simulink model "nuclearReactor"  (R2014b)
settings: Solver=ode1  StartTime=0.0  StopTime=100  FixedStep=0.0001  MaxStep=0.0001  RelTol=1e-3
(part 4 of 4)

== matlab function nuclearReactor/Controller20/MATLAB Function ==
  data: q input; qNext output; x input; r1 output; r2 output; y1 input; y2 input; control output


function [qNext,r1,r2,control]  = phi(q, x, y1, y2)
%#codegen
% control {-1 undefined, 0 add1, 1 remove1, 2 add2, 3 remove2}

undef =0;
add1 = 1;
remove1 =2;
add2 = 3;
remove2 =4;
c=15;

if q==0 
    %When plant is in T0 ("No Rod")
    if x > 550 && y1 >= c && y2<c
        qNext=1;
        r1=0; r2=0;
        control=add1;
    elseif x>550 && y2>=c
        qNext=2;
        r1=0; r2=0;
        control=add2;
    else
        qNext=0;
        r1=0; r2=0;
        control=undef;
    end;
    
elseif q==1    
    %When plant is in T1 ("Rod One")
    if x <= 510 
        qNext=0;
        r1=1; r2=0;
        control=remove1;
    else
        qNext=1;
        r1=0; r2=0;
        control=undef;
    end;

elseif q==2    
    %When plant is in T2 ("Rod Two")
    if x <= 510 
        qNext=0;
        r1=0; r2=1;
        control=remove2;
    else
        qNext=2;
        r1=0; r2=0;
        control=undef;
    end;
else
    qNext=-1; %this should never execute
    r1=0; r2=0; %this should never execute
    control=-1; %this should never execute
end

== matlab function nuclearReactor/Controller21/MATLAB Function ==
  data: q input; qNext output; x input; r1 output; r2 output; y1 input; y2 input; control output


function [qNext,r1,r2,control]  = phi(q, x, y1, y2)
%#codegen
% control {-1 undefined, 0 add1, 1 remove1, 2 add2, 3 remove2}

undef =0;
add1 = 1;
remove1 =2;
add2 = 3;
remove2 =4;
c=15;

if q==0 
    %When plant is in T0 ("No Rod")
    if x > 550 && y1 >= c && y2<c
        qNext=1;
        r1=0; r2=0;
        control=add1;
    elseif x>550 && y2>=c
        qNext=2;
        r1=0; r2=0;
        control=add2;
    else
        qNext=0;
        r1=0; r2=0;
        control=undef;
    end;
    
elseif q==1    
    %When plant is in T1 ("Rod One")
    if x <= 510 
        qNext=0;
        r1=1; r2=0;
        control=remove1;
    else
        qNext=1;
        r1=0; r2=0;
        control=undef;
    end;

elseif q==2    
    %When plant is in T2 ("Rod Two")
    if x <= 510 
        qNext=0;
        r1=0; r2=1;
        control=remove2;
    else
        qNext=2;
        r1=0; r2=0;
        control=undef;
    end;
else
    qNext=-1; %this should never execute
    r1=0; r2=0; %this should never execute
    control=-1; %this should never execute
end

== matlab function nuclearReactor/Controller22/MATLAB Function ==
  data: q input; qNext output; x input; r1 output; r2 output; y1 input; y2 input; control output


function [qNext,r1,r2,control]  = phi(q, x, y1, y2)
%#codegen
% control {-1 undefined, 0 add1, 1 remove1, 2 add2, 3 remove2}

undef =0;
add1 = 1;
remove1 =2;
add2 = 3;
remove2 =4;
c=15;

if q==0 
    %When plant is in T0 ("No Rod")
    if x > 550 && y1 >= c && y2<c
        qNext=1;
        r1=0; r2=0;
        control=add1;
    elseif x>550 && y2>=c
        qNext=2;
        r1=0; r2=0;
        control=add2;
    else
        qNext=0;
        r1=0; r2=0;
        control=undef;
    end;
    
elseif q==1    
    %When plant is in T1 ("Rod One")
    if x <= 510 
        qNext=0;
        r1=1; r2=0;
        control=remove1;
    else
        qNext=1;
        r1=0; r2=0;
        control=undef;
    end;

elseif q==2    
    %When plant is in T2 ("Rod Two")
    if x <= 510 
        qNext=0;
        r1=0; r2=1;
        control=remove2;
    else
        qNext=2;
        r1=0; r2=0;
        control=undef;
    end;
else
    qNext=-1; %this should never execute
    r1=0; r2=0; %this should never execute
    control=-1; %this should never execute
end

== matlab function nuclearReactor/Controller23/MATLAB Function ==
  data: q input; qNext output; x input; r1 output; r2 output; y1 input; y2 input; control output


function [qNext,r1,r2,control]  = phi(q, x, y1, y2)
%#codegen
% control {-1 undefined, 0 add1, 1 remove1, 2 add2, 3 remove2}

undef =0;
add1 = 1;
remove1 =2;
add2 = 3;
remove2 =4;
c=15;

if q==0 
    %When plant is in T0 ("No Rod")
    if x > 550 && y1 >= c && y2<c
        qNext=1;
        r1=0; r2=0;
        control=add1;
    elseif x>550 && y2>=c
        qNext=2;
        r1=0; r2=0;
        control=add2;
    else
        qNext=0;
        r1=0; r2=0;
        control=undef;
    end;
    
elseif q==1    
    %When plant is in T1 ("Rod One")
    if x <= 510 
        qNext=0;
        r1=1; r2=0;
        control=remove1;
    else
        qNext=1;
        r1=0; r2=0;
        control=undef;
    end;

elseif q==2    
    %When plant is in T2 ("Rod Two")
    if x <= 510 
        qNext=0;
        r1=0; r2=1;
        control=remove2;
    else
        qNext=2;
        r1=0; r2=0;
        control=undef;
    end;
else
    qNext=-1; %this should never execute
    r1=0; r2=0; %this should never execute
    control=-1; %this should never execute
end

== matlab function nuclearReactor/Controller24/MATLAB Function ==
  data: q input; qNext output; x input; r1 output; r2 output; y1 input; y2 input; control output


function [qNext,r1,r2,control]  = phi(q, x, y1, y2)
%#codegen
% control {-1 undefined, 0 add1, 1 remove1, 2 add2, 3 remove2}

undef =0;
add1 = 1;
remove1 =2;
add2 = 3;
remove2 =4;
c=15;

if q==0 
    %When plant is in T0 ("No Rod")
    if x > 550 && y1 >= c && y2<c
        qNext=1;
        r1=0; r2=0;
        control=add1;
    elseif x>550 && y2>=c
        qNext=2;
        r1=0; r2=0;
        control=add2;
    else
        qNext=0;
        r1=0; r2=0;
        control=undef;
    end;
    
elseif q==1    
    %When plant is in T1 ("Rod One")
    if x <= 510 
        qNext=0;
        r1=1; r2=0;
        control=remove1;
    else
        qNext=1;
        r1=0; r2=0;
        control=undef;
    end;

elseif q==2    
    %When plant is in T2 ("Rod Two")
    if x <= 510 
        qNext=0;
        r1=0; r2=1;
        control=remove2;
    else
        qNext=2;
        r1=0; r2=0;
        control=undef;
    end;
else
    qNext=-1; %this should never execute
    r1=0; r2=0; %this should never execute
    control=-1; %this should never execute
end

== matlab function nuclearReactor/Controller25/MATLAB Function ==
  data: q input; qNext output; x input; r1 output; r2 output; y1 input; y2 input; control output


function [qNext,r1,r2,control]  = phi(q, x, y1, y2)
%#codegen
% control {-1 undefined, 0 add1, 1 remove1, 2 add2, 3 remove2}

undef =0;
add1 = 1;
remove1 =2;
add2 = 3;
remove2 =4;
c=15;

if q==0 
    %When plant is in T0 ("No Rod")
    if x > 550 && y1 >= c && y2<c
        qNext=1;
        r1=0; r2=0;
        control=add1;
    elseif x>550 && y2>=c
        qNext=2;
        r1=0; r2=0;
        control=add2;
    else
        qNext=0;
        r1=0; r2=0;
        control=undef;
    end;
    
elseif q==1    
    %When plant is in T1 ("Rod One")
    if x <= 510 
        qNext=0;
        r1=1; r2=0;
        control=remove1;
    else
        qNext=1;
        r1=0; r2=0;
        control=undef;
    end;

elseif q==2    
    %When plant is in T2 ("Rod Two")
    if x <= 510 
        qNext=0;
        r1=0; r2=1;
        control=remove2;
    else
        qNext=2;
        r1=0; r2=0;
        control=undef;
    end;
else
    qNext=-1; %this should never execute
    r1=0; r2=0; %this should never execute
    control=-1; %this should never execute
end

== matlab function nuclearReactor/Controller26/MATLAB Function ==
  data: q input; qNext output; x input; r1 output; r2 output; y1 input; y2 input; control output


function [qNext,r1,r2,control]  = phi(q, x, y1, y2)
%#codegen
% control {-1 undefined, 0 add1, 1 remove1, 2 add2, 3 remove2}

undef =0;
add1 = 1;
remove1 =2;
add2 = 3;
remove2 =4;
c=15;

if q==0 
    %When plant is in T0 ("No Rod")
    if x > 550 && y1 >= c && y2<c
        qNext=1;
        r1=0; r2=0;
        control=add1;
    elseif x>550 && y2>=c
        qNext=2;
        r1=0; r2=0;
        control=add2;
    else
        qNext=0;
        r1=0; r2=0;
        control=undef;
    end;
    
elseif q==1    
    %When plant is in T1 ("Rod One")
    if x <= 510 
        qNext=0;
        r1=1; r2=0;
        control=remove1;
    else
        qNext=1;
        r1=0; r2=0;
        control=undef;
    end;

elseif q==2    
    %When plant is in T2 ("Rod Two")
    if x <= 510 
        qNext=0;
        r1=0; r2=1;
        control=remove2;
    else
        qNext=2;
        r1=0; r2=0;
        control=undef;
    end;
else
    qNext=-1; %this should never execute
    r1=0; r2=0; %this should never execute
    control=-1; %this should never execute
end

== matlab function nuclearReactor/Controller27/MATLAB Function ==
  data: q input; qNext output; x input; r1 output; r2 output; y1 input; y2 input; control output


function [qNext,r1,r2,control]  = phi(q, x, y1, y2)
%#codegen
% control {-1 undefined, 0 add1, 1 remove1, 2 add2, 3 remove2}

undef =0;
add1 = 1;
remove1 =2;
add2 = 3;
remove2 =4;
c=15;

if q==0 
    %When plant is in T0 ("No Rod")
    if x > 550 && y1 >= c && y2<c
        qNext=1;
        r1=0; r2=0;
        control=add1;
    elseif x>550 && y2>=c
        qNext=2;
        r1=0; r2=0;
        control=add2;
    else
        qNext=0;
        r1=0; r2=0;
        control=undef;
    end;
    
elseif q==1    
    %When plant is in T1 ("Rod One")
    if x <= 510 
        qNext=0;
        r1=1; r2=0;
        control=remove1;
    else
        qNext=1;
        r1=0; r2=0;
        control=undef;
    end;

elseif q==2    
    %When plant is in T2 ("Rod Two")
    if x <= 510 
        qNext=0;
        r1=0; r2=1;
        control=remove2;
    else
        qNext=2;
        r1=0; r2=0;
        control=undef;
    end;
else
    qNext=-1; %this should never execute
    r1=0; r2=0; %this should never execute
    control=-1; %this should never execute
end

== matlab function nuclearReactor/Controller28/MATLAB Function ==
  data: q input; qNext output; x input; r1 output; r2 output; y1 input; y2 input; control output


function [qNext,r1,r2,control]  = phi(q, x, y1, y2)
%#codegen
% control {-1 undefined, 0 add1, 1 remove1, 2 add2, 3 remove2}

undef =0;
add1 = 1;
remove1 =2;
add2 = 3;
remove2 =4;
c=15;

if q==0 
    %When plant is in T0 ("No Rod")
    if x > 550 && y1 >= c && y2<c
        qNext=1;
        r1=0; r2=0;
        control=add1;
    elseif x>550 && y2>=c
        qNext=2;
        r1=0; r2=0;
        control=add2;
    else
        qNext=0;
        r1=0; r2=0;
        control=undef;
    end;
    
elseif q==1    
    %When plant is in T1 ("Rod One")
    if x <= 510 
        qNext=0;
        r1=1; r2=0;
        control=remove1;
    else
        qNext=1;
        r1=0; r2=0;
        control=undef;
    end;

elseif q==2    
    %When plant is in T2 ("Rod Two")
    if x <= 510 
        qNext=0;
        r1=0; r2=1;
        control=remove2;
    else
        qNext=2;
        r1=0; r2=0;
        control=undef;
    end;
else
    qNext=-1; %this should never execute
    r1=0; r2=0; %this should never execute
    control=-1; %this should never execute
end

== matlab function nuclearReactor/Controller29/MATLAB Function ==
  data: q input; qNext output; x input; r1 output; r2 output; y1 input; y2 input; control output


function [qNext,r1,r2,control]  = phi(q, x, y1, y2)
%#codegen
% control {-1 undefined, 0 add1, 1 remove1, 2 add2, 3 remove2}

undef =0;
add1 = 1;
remove1 =2;
add2 = 3;
remove2 =4;
c=15;

if q==0 
    %When plant is in T0 ("No Rod")
    if x > 550 && y1 >= c && y2<c
        qNext=1;
        r1=0; r2=0;
        control=add1;
    elseif x>550 && y2>=c
        qNext=2;
        r1=0; r2=0;
        control=add2;
    else
        qNext=0;
        r1=0; r2=0;
        control=undef;
    end;
    
elseif q==1    
    %When plant is in T1 ("Rod One")
    if x <= 510 
        qNext=0;
        r1=1; r2=0;
        control=remove1;
    else
        qNext=1;
        r1=0; r2=0;
        control=undef;
    end;

elseif q==2    
    %When plant is in T2 ("Rod Two")
    if x <= 510 
        qNext=0;
        r1=0; r2=1;
        control=remove2;
    else
        qNext=2;
        r1=0; r2=0;
        control=undef;
    end;
else
    qNext=-1; %this should never execute
    r1=0; r2=0; %this should never execute
    control=-1; %this should never execute
end

== matlab function nuclearReactor/Plant15/MATLAB Function ==
  data: q input; qNext output; control input; reset output


function [qNext,reset]  = phi(q, control)
%#codegen
% control {-1 undefined, 0 add1, 1 remove1, 2 add2, 3 remove2}

undef =0;
add1 = 1;
remove1 =2;
add2 = 3;
remove2 =4;
c=10;

if q==0 
    %When plant is in T0 ("No Rod")
    if control ==add1
        qNext=1;
        reset=1;
    elseif control ==add2
        qNext=2;
        reset=1;
    else
        qNext=0;
        reset=0;
    end;
    
elseif q==1    
    %When plant is in T1 ("Rod One")
    if control ==remove1
        qNext=0;
        reset=1;
    else
        qNext=1;
        reset=0;
    end;

elseif q==2    
    %When plant is in T2 ("Rod Two")
    if control ==remove2
        qNext=0;
        reset=1;
    else
        qNext=2;
        reset=0;
    end;
else
    qNext=-1; %this should never execute
    reset=-1; %this should never execute
end

== matlab function nuclearReactor/Plant15/MATLAB Function1 ==
  data: x input; x_dot0 output; x_dot1 output; x_dot2 output
function [x_dot0, x_dot1, x_dot2] = ODEs(x)
%#codegen
x_dot0=0.1*x-50;
x_dot1=0.1*x-56;
x_dot2=0.1*x-60;

== matlab function nuclearReactor/Plant16/MATLAB Function ==
  data: q input; qNext output; control input; reset output


function [qNext,reset]  = phi(q, control)
%#codegen
% control {-1 undefined, 0 add1, 1 remove1, 2 add2, 3 remove2}

undef =0;
add1 = 1;
remove1 =2;
add2 = 3;
remove2 =4;
c=10;

if q==0 
    %When plant is in T0 ("No Rod")
    if control ==add1
        qNext=1;
        reset=1;
    elseif control ==add2
        qNext=2;
        reset=1;
    else
        qNext=0;
        reset=0;
    end;
    
elseif q==1    
    %When plant is in T1 ("Rod One")
    if control ==remove1
        qNext=0;
        reset=1;
    else
        qNext=1;
        reset=0;
    end;

elseif q==2    
    %When plant is in T2 ("Rod Two")
    if control ==remove2
        qNext=0;
        reset=1;
    else
        qNext=2;
        reset=0;
    end;
else
    qNext=-1; %this should never execute
    reset=-1; %this should never execute
end

== matlab function nuclearReactor/Plant16/MATLAB Function1 ==
  data: x input; x_dot0 output; x_dot1 output; x_dot2 output
function [x_dot0, x_dot1, x_dot2] = ODEs(x)
%#codegen
x_dot0=0.1*x-50;
x_dot1=0.1*x-56;
x_dot2=0.1*x-60;

== matlab function nuclearReactor/Plant17/MATLAB Function ==
  data: q input; qNext output; control input; reset output


function [qNext,reset]  = phi(q, control)
%#codegen
% control {-1 undefined, 0 add1, 1 remove1, 2 add2, 3 remove2}

undef =0;
add1 = 1;
remove1 =2;
add2 = 3;
remove2 =4;
c=10;

if q==0 
    %When plant is in T0 ("No Rod")
    if control ==add1
        qNext=1;
        reset=1;
    elseif control ==add2
        qNext=2;
        reset=1;
    else
        qNext=0;
        reset=0;
    end;
    
elseif q==1    
    %When plant is in T1 ("Rod One")
    if control ==remove1
        qNext=0;
        reset=1;
    else
        qNext=1;
        reset=0;
    end;

elseif q==2    
    %When plant is in T2 ("Rod Two")
    if control ==remove2
        qNext=0;
        reset=1;
    else
        qNext=2;
        reset=0;
    end;
else
    qNext=-1; %this should never execute
    reset=-1; %this should never execute
end

== matlab function nuclearReactor/Plant17/MATLAB Function1 ==
  data: x input; x_dot0 output; x_dot1 output; x_dot2 output
function [x_dot0, x_dot1, x_dot2] = ODEs(x)
%#codegen
x_dot0=0.1*x-50;
x_dot1=0.1*x-56;
x_dot2=0.1*x-60;

== matlab function nuclearReactor/Plant18/MATLAB Function ==
  data: q input; qNext output; control input; reset output


function [qNext,reset]  = phi(q, control)
%#codegen
% control {-1 undefined, 0 add1, 1 remove1, 2 add2, 3 remove2}

undef =0;
add1 = 1;
remove1 =2;
add2 = 3;
remove2 =4;
c=10;

if q==0 
    %When plant is in T0 ("No Rod")
    if control ==add1
        qNext=1;
        reset=1;
    elseif control ==add2
        qNext=2;
        reset=1;
    else
        qNext=0;
        reset=0;
    end;
    
elseif q==1    
    %When plant is in T1 ("Rod One")
    if control ==remove1
        qNext=0;
        reset=1;
    else
        qNext=1;
        reset=0;
    end;

elseif q==2    
    %When plant is in T2 ("Rod Two")
    if control ==remove2
        qNext=0;
        reset=1;
    else
        qNext=2;
        reset=0;
    end;
else
    qNext=-1; %this should never execute
    reset=-1; %this should never execute
end

== matlab function nuclearReactor/Plant18/MATLAB Function1 ==
  data: x input; x_dot0 output; x_dot1 output; x_dot2 output
function [x_dot0, x_dot1, x_dot2] = ODEs(x)
%#codegen
x_dot0=0.1*x-50;
x_dot1=0.1*x-56;
x_dot2=0.1*x-60;

== matlab function nuclearReactor/Plant19/MATLAB Function ==
  data: q input; qNext output; control input; reset output


function [qNext,reset]  = phi(q, control)
%#codegen
% control {-1 undefined, 0 add1, 1 remove1, 2 add2, 3 remove2}

undef =0;
add1 = 1;
remove1 =2;
add2 = 3;
remove2 =4;
c=10;

if q==0 
    %When plant is in T0 ("No Rod")
    if control ==add1
        qNext=1;
        reset=1;
    elseif control ==add2
        qNext=2;
        reset=1;
    else
        qNext=0;
        reset=0;
    end;
    
elseif q==1    
    %When plant is in T1 ("Rod One")
    if control ==remove1
        qNext=0;
        reset=1;
    else
        qNext=1;
        reset=0;
    end;

elseif q==2    
    %When plant is in T2 ("Rod Two")
    if control ==remove2
        qNext=0;
        reset=1;
    else
        qNext=2;
        reset=0;
    end;
else
    qNext=-1; %this should never execute
    reset=-1; %this should never execute
end

== matlab function nuclearReactor/Plant19/MATLAB Function1 ==
  data: x input; x_dot0 output; x_dot1 output; x_dot2 output
function [x_dot0, x_dot1, x_dot2] = ODEs(x)
%#codegen
x_dot0=0.1*x-50;
x_dot1=0.1*x-56;
x_dot2=0.1*x-60;

== matlab function nuclearReactor/Plant20/MATLAB Function ==
  data: q input; qNext output; control input; reset output


function [qNext,reset]  = phi(q, control)
%#codegen
% control {-1 undefined, 0 add1, 1 remove1, 2 add2, 3 remove2}

undef =0;
add1 = 1;
remove1 =2;
add2 = 3;
remove2 =4;
c=10;

if q==0 
    %When plant is in T0 ("No Rod")
    if control ==add1
        qNext=1;
        reset=1;
    elseif control ==add2
        qNext=2;
        reset=1;
    else
        qNext=0;
        reset=0;
    end;
    
elseif q==1    
    %When plant is in T1 ("Rod One")
    if control ==remove1
        qNext=0;
        reset=1;
    else
        qNext=1;
        reset=0;
    end;

elseif q==2    
    %When plant is in T2 ("Rod Two")
    if control ==remove2
        qNext=0;
        reset=1;
    else
        qNext=2;
        reset=0;
    end;
else
    qNext=-1; %this should never execute
    reset=-1; %this should never execute
end

== matlab function nuclearReactor/Plant20/MATLAB Function1 ==
  data: x input; x_dot0 output; x_dot1 output; x_dot2 output
function [x_dot0, x_dot1, x_dot2] = ODEs(x)
%#codegen
x_dot0=0.1*x-50;
x_dot1=0.1*x-56;
x_dot2=0.1*x-60;

== matlab function nuclearReactor/Plant21/MATLAB Function ==
  data: q input; qNext output; control input; reset output


function [qNext,reset]  = phi(q, control)
%#codegen
% control {-1 undefined, 0 add1, 1 remove1, 2 add2, 3 remove2}

undef =0;
add1 = 1;
remove1 =2;
add2 = 3;
remove2 =4;
c=10;

if q==0 
    %When plant is in T0 ("No Rod")
    if control ==add1
        qNext=1;
        reset=1;
    elseif control ==add2
        qNext=2;
        reset=1;
    else
        qNext=0;
        reset=0;
    end;
    
elseif q==1    
    %When plant is in T1 ("Rod One")
    if control ==remove1
        qNext=0;
        reset=1;
    else
        qNext=1;
        reset=0;
    end;

elseif q==2    
    %When plant is in T2 ("Rod Two")
    if control ==remove2
        qNext=0;
        reset=1;
    else
        qNext=2;
        reset=0;
    end;
else
    qNext=-1; %this should never execute
    reset=-1; %this should never execute
end

== matlab function nuclearReactor/Plant21/MATLAB Function1 ==
  data: x input; x_dot0 output; x_dot1 output; x_dot2 output
function [x_dot0, x_dot1, x_dot2] = ODEs(x)
%#codegen
x_dot0=0.1*x-50;
x_dot1=0.1*x-56;
x_dot2=0.1*x-60;

== matlab function nuclearReactor/Plant22/MATLAB Function ==
  data: q input; qNext output; control input; reset output


function [qNext,reset]  = phi(q, control)
%#codegen
% control {-1 undefined, 0 add1, 1 remove1, 2 add2, 3 remove2}

undef =0;
add1 = 1;
remove1 =2;
add2 = 3;
remove2 =4;
c=10;

if q==0 
    %When plant is in T0 ("No Rod")
    if control ==add1
        qNext=1;
        reset=1;
    elseif control ==add2
        qNext=2;
        reset=1;
    else
        qNext=0;
        reset=0;
    end;
    
elseif q==1    
    %When plant is in T1 ("Rod One")
    if control ==remove1
        qNext=0;
        reset=1;
    else
        qNext=1;
        reset=0;
    end;

elseif q==2    
    %When plant is in T2 ("Rod Two")
    if control ==remove2
        qNext=0;
        reset=1;
    else
        qNext=2;
        reset=0;
    end;
else
    qNext=-1; %this should never execute
    reset=-1; %this should never execute
end

== matlab function nuclearReactor/Plant22/MATLAB Function1 ==
  data: x input; x_dot0 output; x_dot1 output; x_dot2 output
function [x_dot0, x_dot1, x_dot2] = ODEs(x)
%#codegen
x_dot0=0.1*x-50;
x_dot1=0.1*x-56;
x_dot2=0.1*x-60;

== matlab function nuclearReactor/Plant23/MATLAB Function ==
  data: q input; qNext output; control input; reset output


function [qNext,reset]  = phi(q, control)
%#codegen
% control {-1 undefined, 0 add1, 1 remove1, 2 add2, 3 remove2}

undef =0;
add1 = 1;
remove1 =2;
add2 = 3;
remove2 =4;
c=10;

if q==0 
    %When plant is in T0 ("No Rod")
    if control ==add1
        qNext=1;
        reset=1;
    elseif control ==add2
        qNext=2;
        reset=1;
    else
        qNext=0;
        reset=0;
    end;
    
elseif q==1    
    %When plant is in T1 ("Rod One")
    if control ==remove1
        qNext=0;
        reset=1;
    else
        qNext=1;
        reset=0;
    end;

elseif q==2    
    %When plant is in T2 ("Rod Two")
    if control ==remove2
        qNext=0;
        reset=1;
    else
        qNext=2;
        reset=0;
    end;
else
    qNext=-1; %this should never execute
    reset=-1; %this should never execute
end

== matlab function nuclearReactor/Plant23/MATLAB Function1 ==
  data: x input; x_dot0 output; x_dot1 output; x_dot2 output
function [x_dot0, x_dot1, x_dot2] = ODEs(x)
%#codegen
x_dot0=0.1*x-50;
x_dot1=0.1*x-56;
x_dot2=0.1*x-60;

== matlab function nuclearReactor/Plant24/MATLAB Function ==
  data: q input; qNext output; control input; reset output


function [qNext,reset]  = phi(q, control)
%#codegen
% control {-1 undefined, 0 add1, 1 remove1, 2 add2, 3 remove2}

undef =0;
add1 = 1;
remove1 =2;
add2 = 3;
remove2 =4;
c=10;

if q==0 
    %When plant is in T0 ("No Rod")
    if control ==add1
        qNext=1;
        reset=1;
    elseif control ==add2
        qNext=2;
        reset=1;
    else
        qNext=0;
        reset=0;
    end;
    
elseif q==1    
    %When plant is in T1 ("Rod One")
    if control ==remove1
        qNext=0;
        reset=1;
    else
        qNext=1;
        reset=0;
    end;

elseif q==2    
    %When plant is in T2 ("Rod Two")
    if control ==remove2
        qNext=0;
        reset=1;
    else
        qNext=2;
        reset=0;
    end;
else
    qNext=-1; %this should never execute
    reset=-1; %this should never execute
end

== matlab function nuclearReactor/Plant24/MATLAB Function1 ==
  data: x input; x_dot0 output; x_dot1 output; x_dot2 output
function [x_dot0, x_dot1, x_dot2] = ODEs(x)
%#codegen
x_dot0=0.1*x-50;
x_dot1=0.1*x-56;
x_dot2=0.1*x-60;

== matlab function nuclearReactor/Plant25/MATLAB Function ==
  data: q input; qNext output; control input; reset output


function [qNext,reset]  = phi(q, control)
%#codegen
% control {-1 undefined, 0 add1, 1 remove1, 2 add2, 3 remove2}

undef =0;
add1 = 1;
remove1 =2;
add2 = 3;
remove2 =4;
c=10;

if q==0 
    %When plant is in T0 ("No Rod")
    if control ==add1
        qNext=1;
        reset=1;
    elseif control ==add2
        qNext=2;
        reset=1;
    else
        qNext=0;
        reset=0;
    end;
    
elseif q==1    
    %When plant is in T1 ("Rod One")
    if control ==remove1
        qNext=0;
        reset=1;
    else
        qNext=1;
        reset=0;
    end;

elseif q==2    
    %When plant is in T2 ("Rod Two")
    if control ==remove2
        qNext=0;
        reset=1;
    else
        qNext=2;
        reset=0;
    end;
else
    qNext=-1; %this should never execute
    reset=-1; %this should never execute
end

== matlab function nuclearReactor/Plant25/MATLAB Function1 ==
  data: x input; x_dot0 output; x_dot1 output; x_dot2 output
function [x_dot0, x_dot1, x_dot2] = ODEs(x)
%#codegen
x_dot0=0.1*x-50;
x_dot1=0.1*x-56;
x_dot2=0.1*x-60;

== matlab function nuclearReactor/Plant26/MATLAB Function ==
  data: q input; qNext output; control input; reset output


function [qNext,reset]  = phi(q, control)
%#codegen
% control {-1 undefined, 0 add1, 1 remove1, 2 add2, 3 remove2}

undef =0;
add1 = 1;
remove1 =2;
add2 = 3;
remove2 =4;
c=10;

if q==0 
    %When plant is in T0 ("No Rod")
    if control ==add1
        qNext=1;
        reset=1;
    elseif control ==add2
        qNext=2;
        reset=1;
    else
        qNext=0;
        reset=0;
    end;
    
elseif q==1    
    %When plant is in T1 ("Rod One")
    if control ==remove1
        qNext=0;
        reset=1;
    else
        qNext=1;
        reset=0;
    end;

elseif q==2    
    %When plant is in T2 ("Rod Two")
    if control ==remove2
        qNext=0;
        reset=1;
    else
        qNext=2;
        reset=0;
    end;
else
    qNext=-1; %this should never execute
    reset=-1; %this should never execute
end

== matlab function nuclearReactor/Plant26/MATLAB Function1 ==
  data: x input; x_dot0 output; x_dot1 output; x_dot2 output
function [x_dot0, x_dot1, x_dot2] = ODEs(x)
%#codegen
x_dot0=0.1*x-50;
x_dot1=0.1*x-56;
x_dot2=0.1*x-60;

== matlab function nuclearReactor/Plant27/MATLAB Function ==
  data: q input; qNext output; control input; reset output


function [qNext,reset]  = phi(q, control)
%#codegen
% control {-1 undefined, 0 add1, 1 remove1, 2 add2, 3 remove2}

undef =0;
add1 = 1;
remove1 =2;
add2 = 3;
remove2 =4;
c=10;

if q==0 
    %When plant is in T0 ("No Rod")
    if control ==add1
        qNext=1;
        reset=1;
    elseif control ==add2
        qNext=2;
        reset=1;
    else
        qNext=0;
        reset=0;
    end;
    
elseif q==1    
    %When plant is in T1 ("Rod One")
    if control ==remove1
        qNext=0;
        reset=1;
    else
        qNext=1;
        reset=0;
    end;

elseif q==2    
    %When plant is in T2 ("Rod Two")
    if control ==remove2
        qNext=0;
        reset=1;
    else
        qNext=2;
        reset=0;
    end;
else
    qNext=-1; %this should never execute
    reset=-1; %this should never execute
end

== matlab function nuclearReactor/Plant27/MATLAB Function1 ==
  data: x input; x_dot0 output; x_dot1 output; x_dot2 output
function [x_dot0, x_dot1, x_dot2] = ODEs(x)
%#codegen
x_dot0=0.1*x-50;
x_dot1=0.1*x-56;
x_dot2=0.1*x-60;

== matlab function nuclearReactor/Plant28/MATLAB Function ==
  data: q input; qNext output; control input; reset output


function [qNext,reset]  = phi(q, control)
%#codegen
% control {-1 undefined, 0 add1, 1 remove1, 2 add2, 3 remove2}

undef =0;
add1 = 1;
remove1 =2;
add2 = 3;
remove2 =4;
c=10;

if q==0 
    %When plant is in T0 ("No Rod")
    if control ==add1
        qNext=1;
        reset=1;
    elseif control ==add2
        qNext=2;
        reset=1;
    else
        qNext=0;
        reset=0;
    end;
    
elseif q==1    
    %When plant is in T1 ("Rod One")
    if control ==remove1
        qNext=0;
        reset=1;
    else
        qNext=1;
        reset=0;
    end;

elseif q==2    
    %When plant is in T2 ("Rod Two")
    if control ==remove2
        qNext=0;
        reset=1;
    else
        qNext=2;
        reset=0;
    end;
else
    qNext=-1; %this should never execute
    reset=-1; %this should never execute
end

== matlab function nuclearReactor/Plant28/MATLAB Function1 ==
  data: x input; x_dot0 output; x_dot1 output; x_dot2 output
function [x_dot0, x_dot1, x_dot2] = ODEs(x)
%#codegen
x_dot0=0.1*x-50;
x_dot1=0.1*x-56;
x_dot2=0.1*x-60;

== matlab function nuclearReactor/Plant29/MATLAB Function ==
  data: q input; qNext output; control input; reset output


function [qNext,reset]  = phi(q, control)
%#codegen
% control {-1 undefined, 0 add1, 1 remove1, 2 add2, 3 remove2}

undef =0;
add1 = 1;
remove1 =2;
add2 = 3;
remove2 =4;
c=10;

if q==0 
    %When plant is in T0 ("No Rod")
    if control ==add1
        qNext=1;
        reset=1;
    elseif control ==add2
        qNext=2;
        reset=1;
    else
        qNext=0;
        reset=0;
    end;
    
elseif q==1    
    %When plant is in T1 ("Rod One")
    if control ==remove1
        qNext=0;
        reset=1;
    else
        qNext=1;
        reset=0;
    end;

elseif q==2    
    %When plant is in T2 ("Rod Two")
    if control ==remove2
        qNext=0;
        reset=1;
    else
        qNext=2;
        reset=0;
    end;
else
    qNext=-1; %this should never execute
    reset=-1; %this should never execute
end

== matlab function nuclearReactor/Plant29/MATLAB Function1 ==
  data: x input; x_dot0 output; x_dot1 output; x_dot2 output
function [x_dot0, x_dot1, x_dot2] = ODEs(x)
%#codegen
x_dot0=0.1*x-50;
x_dot1=0.1*x-56;
x_dot2=0.1*x-60;
